simulink model "model"  (R2023b)
settings: Solver=FixedStepAuto  StartTime=0.0  StopTime=10.0  FixedStep=0.001  RelTol=1e-3
values from neighbouring files (symbols this model uses):
  amp = 1    [matlab_data.m]
  bias = 1    [matlab_data.m]
  freq = 1    [matlab_data.m]
  phase = 1    [matlab_data.m]
libraries: instrumentseriallib x3
settings Model: Creator=deniskirbaba  LastModifiedBy=deniskirbaba

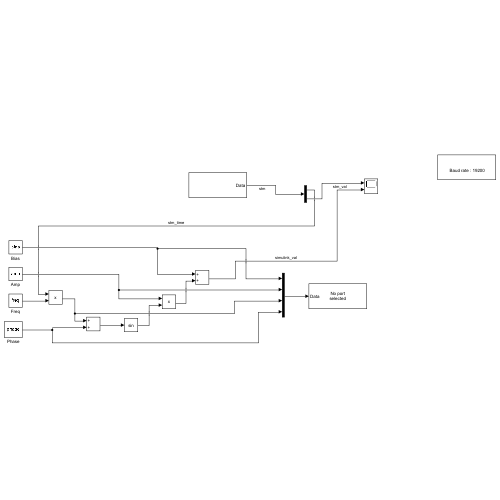
[thumbnail: Simulink's stored preview of the top-level diagram]
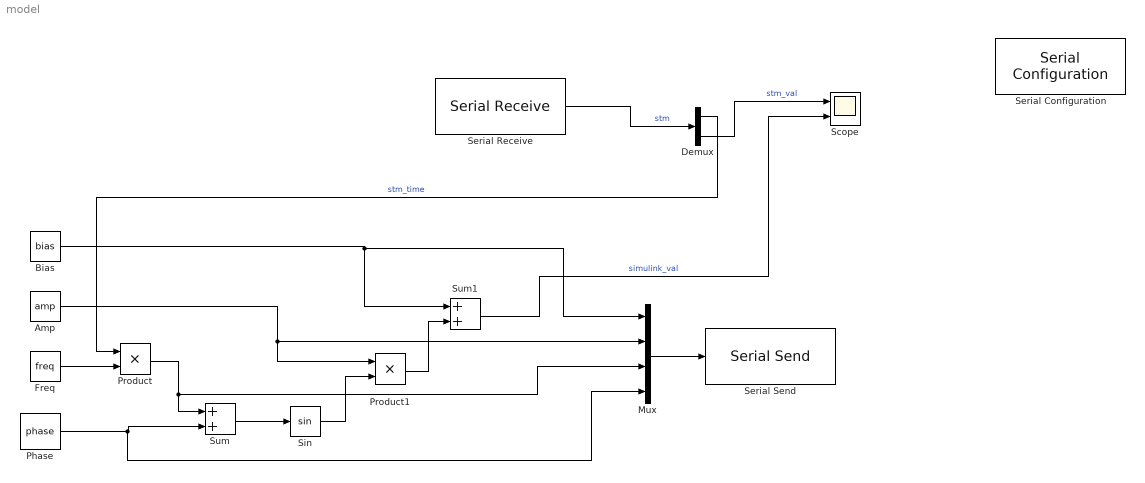
== system model ==
  Amp : Constant  Value=amp
  Bias : Constant  Value=bias
  Demux : Demux  Outputs=2
  Freq : Constant  Value=freq
  Mux : Mux
  Phase : Constant  Value=phase
  Product : Product
  Product1 : Product
  Scope : Scope  NumInputPorts=2
  Serial Configuration : instrumentseriallib/Serial Configuration  Priority=-200000  BaudRate=19200  DataBits=8  Parity=none  StopBits=1  ByteOrder=little-endian  FlowControl=none  Timeout=10  SimulateUsing=Interpreted execution  BlockInModel=on  aMode=1
  Serial Receive : instrumentseriallib/Serial Receive  Priority=1  DataType=single  SaveDataType=uint8  ToggleHeader=on  Header=[78]  ToggleTerminator=on  Terminator=Custom terminator  CustomTerminator=[69]  InputFormat=Column major  ToggleDataSize=on  DataSize=[2 1]  EnableBlockingMode=on  ActionDataUnavailable=Output custom value  ActionWhenDataUnavailable=Output custom value  CustomValue=0  SampleTime=0.01  SimulateUsing=Interpreted execution  BlockInModel=on  aMode=1
  Serial Send : instrumentseriallib/Serial Send  Priority=1  PortSel=<Select a port...>  Port=<Select a port...>  ComPort=<Select a port...>  Header=[78]  Terminator=Custom terminator  CustomTerminator=[69]  EnableBlockingMode=on  SimulateUsing=Interpreted execution  BlockInModel=on  aMode=1
  Sin : Trigonometry
  Sum : Sum
  Sum1 : Sum
  wires:
  Demux/1 -> Product/1  "stm_time"
  Freq/1 -> Product/2
  Phase/1 -> Mux/4, Sum/2
  Product/1 -> Mux/3, Sum/1
  Sum/1 -> Sin/1
  Sin/1 -> Product1/2
  Amp/1 -> Mux/2, Product1/1
  Product1/1 -> Sum1/2
  Bias/1 -> Mux/1, Sum1/1
  Sum1/1 -> Scope/2  "simulink_val"
  Mux/1 -> Serial Send/1
  Serial Receive/1 -> Demux/1  "stm"
  Demux/2 -> Scope/1  "stm_val"
